simulink model "FPGADataCapture_model"  (R2024a)
settings: Solver=VariableStepAuto  StartTime=0.0  StopTime=127  RelTol=1e-3
libraries: hdlverifier_fpga_reader x1
settings Model: Creator=cotti  LastModifiedBy=cotti

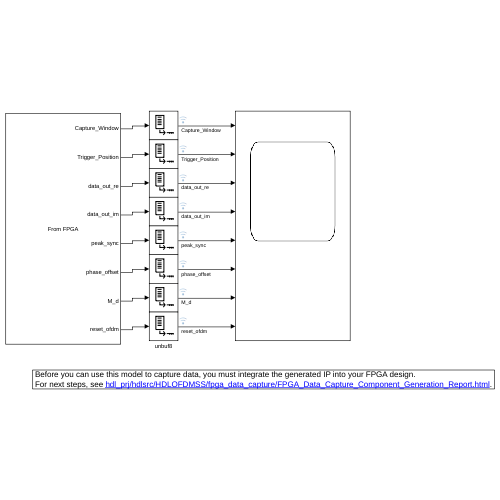
[thumbnail: Simulink's stored preview of the top-level diagram]
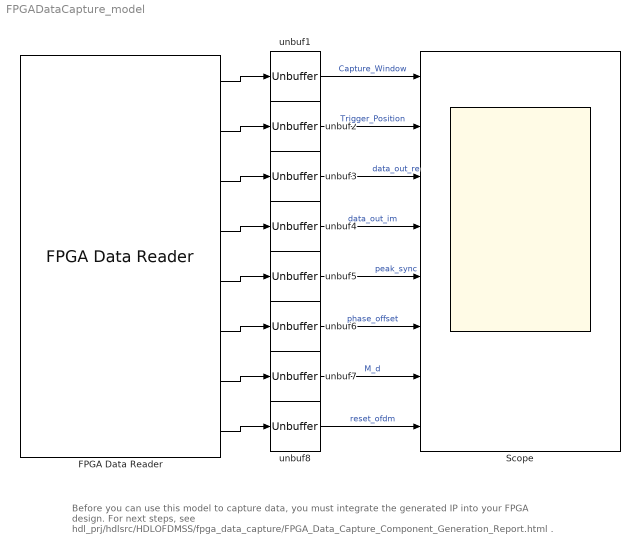
== system FPGADataCapture_model ==
  note: Before you can use this model to capture data, you must integrate the generated IP into your FPGA design.
      | For next steps, see hdl_prj/hdlsrc/HDLOFDMSS/fpga_data_capture/FPGA_Data_Capture_Component_Generation_Report.html .
  FPGA Data Reader : hdlverifier_fpga_reader/FPGA Data Reader  SampleTime=128  FPGAVendor=Xilinx  SamplesPerFrame=128  TriggerPosition=0  NumCaptureWindows=1  MaxNumTriggerStages=1  NumTriggerStages=1  Connection=JTAG  EthInterface=GMII  TimeOut=10  TriggerConditionStr="[false,\"0\",\"==\",0,false,\"0\",\"==\",0,false,\"Low\",\"==\",0,false,\"0\",\"==\",0,false,\"0\",\"==\",0,false,\"Low\",\"==\",0,\"and\",0,1]"  DataTypeStr="[\"uint32\",\"boolean\",\"numerictype(1,16,14)\",\"numerictype(1,16,14)\",\"boolean\",\"numerictype(1,16,15)\",\"numerictype(1,16,14)\",\"boolean\"]"  BitWidth="[32   1  16  16   1  16  16   1]"  SignalNames={'Capture_Window','Trigger_Position','data_out_re','data_out_im','peak_sync','phase_offset','M_d','reset_ofdm'}  IsSignalTrigger="[0  0  1  1  1  1  1  1]"  IsSignalData="[0  0  1  1  1  1  1  1]"  IsMetaData="[1  1  0  0  0  0  0  0]"  RunImmediately=false  CaptureConditionStr="[false,\"0\",\"==\",0,false,\"0\",\"==\",0,false,\"Low\",\"==\",0,false,\"0\",\"==\",0,false,\"0\",\"==\",0,false,\"Low\",\"==\",0,\"and\"]"  IsConditionalCapture=0  DataCaptureName=datacapture1  EnableCaptureCtrl=false  DataCaptureID=1  JTAGCableName=auto  JTAGCableType=auto  JTAGChainPosition=0  IRLengthBefore=0  IRLengthAfter=0  TckFrequency=15  DeviceAddress=192.168.0.2  Port=50101  CaptureBaseAddress=40000000
  Scope : Scope  NumInputPorts=8
  unbuf{1..8} (8 alike) : Unbuffer
  wires:
  FPGA Data Reader/1 -> unbuf1/1
  unbuf1/1 -> Scope/1  "Capture_Window"
  FPGA Data Reader/2 -> unbuf2/1
  unbuf2/1 -> Scope/2  "Trigger_Position"
  FPGA Data Reader/3 -> unbuf3/1
  unbuf3/1 -> Scope/3  "data_out_re"
  FPGA Data Reader/4 -> unbuf4/1
  unbuf4/1 -> Scope/4  "data_out_im"
  FPGA Data Reader/5 -> unbuf5/1
  unbuf5/1 -> Scope/5  "peak_sync"
  FPGA Data Reader/6 -> unbuf6/1
  unbuf6/1 -> Scope/6  "phase_offset"
  FPGA Data Reader/7 -> unbuf7/1
  unbuf7/1 -> Scope/7  "M_d"
  FPGA Data Reader/8 -> unbuf8/1
  unbuf8/1 -> Scope/8  "reset_ofdm"
